simulink model "caishi1_3"  (R2022b)
settings: Solver=VariableStepAuto  StartTime=0.0  StopTime=100  RelTol=1e-3
values from neighbouring files (symbols this model uses):
  C = [1 0 0]    [caishi.m]
settings Model: Creator=HONOR  LastModifiedBy=acer
settings DebuggingCC: UnconnectedInputMsg=warning  UnconnectedOutputMsg=warning  UnconnectedLineMsg=warning
settings ModelReferenceCC: EnableRefExpFcnMdlSchedulingChecks=on
settings RTWCC: DLArmComputeVersion=19.05

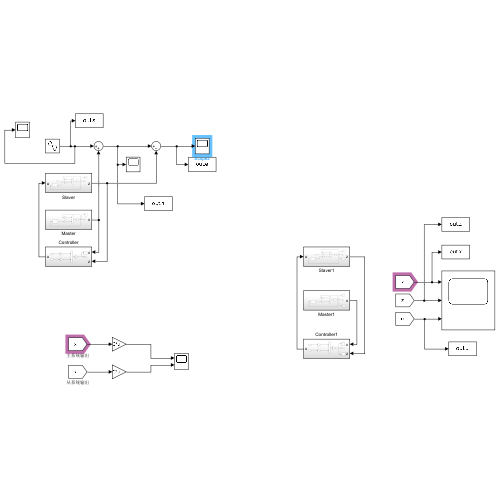
[thumbnail: Simulink's stored preview of the top-level diagram]
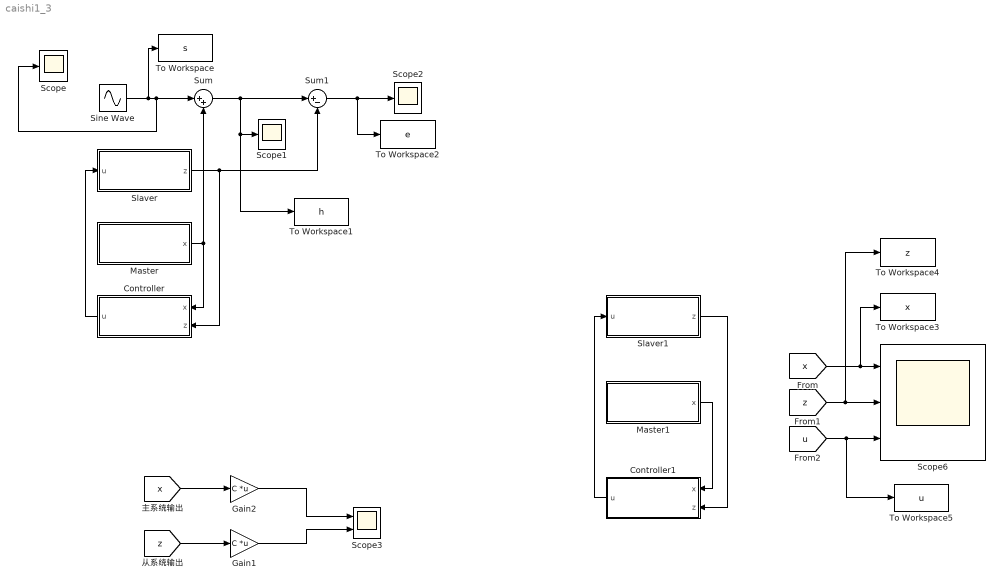
== system caishi1_3 ==
  Controller : Subsystem
  Controller1 : Subsystem
  Gain1 : Gain  Gain=C  Multiplication=Matrix(K*u)
  Gain2 : Gain  Gain=C  Multiplication=Matrix(K*u)
  Master : Subsystem
  Master1 : Subsystem
  Scope : Scope
  Scope1 : Scope
  Scope2 : Scope
  Scope3 : Scope  NumInputPorts=2
  Scope6 : Scope  NumInputPorts=3
  Sine Wave : Sin  SampleTime=0
  Slaver : Subsystem
  Slaver1 : Subsystem
  Sum : Sum  Inputs=|++
  Sum1 : Sum  Inputs=|+-
  To Workspace : ToWorkspace  VariableName=s  SaveFormat=Structure With Time  SampleTime=-1
  To Workspace1 : ToWorkspace  VariableName=h  SaveFormat=Structure With Time  SampleTime=-1
  To Workspace2 : ToWorkspace  VariableName=e  SaveFormat=Structure With Time  SampleTime=-1
  To Workspace3 : ToWorkspace  VariableName=x  SaveFormat=Structure With Time  SampleTime=-1
  To Workspace4 : ToWorkspace  VariableName=z  SaveFormat=Structure With Time  SampleTime=-1
  To Workspace5 : ToWorkspace  VariableName=u  SaveFormat=Structure With Time  SampleTime=-1
  wires:
  Controller/1(u) -> Slaver/1(u)
  Master/1(x) -> Controller/1(x), Sum/2
  Slaver/1(z) -> Sum1/2, Controller/2(z)
  Sine Wave/1 -> To Workspace/1, Scope/1, Sum/1
  Sum/1 -> Sum1/1, To Workspace1/1, Scope1/1
  Sum1/1 -> Scope2/1, To Workspace2/1
  Controller1/1(u) -> Slaver1/1(u)
  Master1/1(x) -> Controller1/1(x)
  Slaver1/1(z) -> Controller1/2(z)
  [z] -> To Workspace4/1, Scope6/2
  [u] -> To Workspace5/1, Scope6/3
  [x] -> To Workspace3/1, Scope6/1
  [x] -> Gain2/1
  [z] -> Gain1/1
  Gain2/1 -> Scope3/1
  Gain1/1 -> Scope3/2

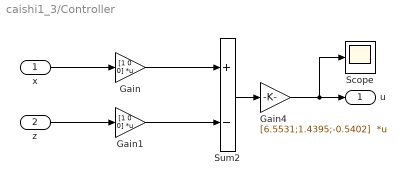
== system caishi1_3/Controller ==
  x : Inport
  z : Inport  Port=2
  Gain : Gain  Gain=[1 0 0]  Multiplication=Matrix(K*u)
  Gain1 : Gain  Gain=[1 0 0]  Multiplication=Matrix(K*u)
  Gain4 : Gain  Gain=[6.5531;1.4395;-0.5402]  Multiplication=Matrix(K*u)
  Scope : Scope
  Sum2 : Sum  Inputs=+-
  u : Outport
  wires:
  Gain1/1 -> Sum2/2
  Gain/1 -> Sum2/1
  Sum2/1 -> Gain4/1
  Gain4/1 -> Scope/1, u/1
  x/1 -> Gain/1
  z/1 -> Gain1/1

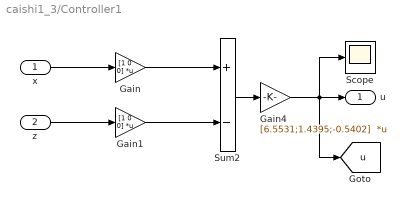
== system caishi1_3/Controller1 ==
  x : Inport
  z : Inport  Port=2
  Gain : Gain  Gain=[1 0 0]  Multiplication=Matrix(K*u)
  Gain1 : Gain  Gain=[1 0 0]  Multiplication=Matrix(K*u)
  Gain4 : Gain  Gain=[6.5531;1.4395;-0.5402]  Multiplication=Matrix(K*u)
  Scope : Scope
  Sum2 : Sum  Inputs=+-
  u : Outport
  tag scope: u=global
  wires:
  Gain1/1 -> Sum2/2
  Gain/1 -> Sum2/1
  Sum2/1 -> Gain4/1
  Gain4/1 -> [u], Scope/1, u/1
  x/1 -> Gain/1
  z/1 -> Gain1/1

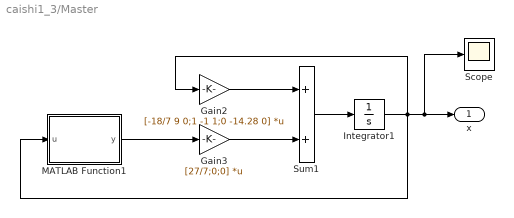
== system caishi1_3/Master ==
  Gain2 : Gain  Gain=[-18/7 9 0;1 -1 1;0 -14.28 0]  Multiplication=Matrix(K*u)
  Gain3 : Gain  Gain=[27/7;0;0]  Multiplication=Matrix(K*u)
  Integrator1 : Integrator  InitialCondition=[-0.1,0.1,0.2]
  MATLAB Function1 : MATLAB Function  TreatAsAtomicUnit=on
  Scope : Scope
  Sum1 : Sum
  x : Outport
  wires:
  Sum1/1 -> Integrator1/1
  Integrator1/1 -> Gain2/1, MATLAB Function1/1(u), Scope/1, x/1
  Gain2/1 -> Sum1/1
  Gain3/1 -> Sum1/2
  MATLAB Function1/1(y) -> Gain3/1

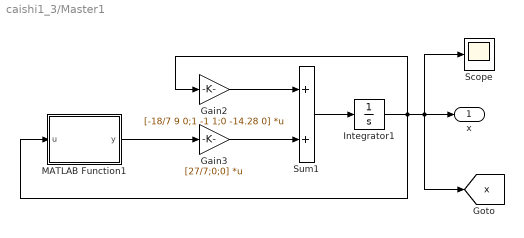
== system caishi1_3/Master1 ==
  Gain2 : Gain  Gain=[-18/7 9 0;1 -1 1;0 -14.28 0]  Multiplication=Matrix(K*u)
  Gain3 : Gain  Gain=[27/7;0;0]  Multiplication=Matrix(K*u)
  Integrator1 : Integrator  InitialCondition=[-0.1,0.1,0.2]
  MATLAB Function1 : MATLAB Function  TreatAsAtomicUnit=on
  Scope : Scope
  Sum1 : Sum
  x : Outport
  tag scope: x=global
  wires:
  Sum1/1 -> Integrator1/1
  Integrator1/1 -> Gain2/1, MATLAB Function1/1(u), [x], Scope/1, x/1
  Gain2/1 -> Sum1/1
  Gain3/1 -> Sum1/2
  MATLAB Function1/1(y) -> Gain3/1

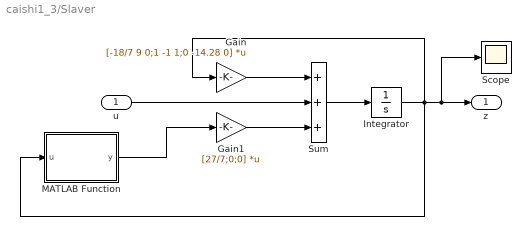
== system caishi1_3/Slaver ==
  u : Inport
  Gain : Gain  Gain=[-18/7 9 0;1 -1 1;0 -14.28 0]  Multiplication=Matrix(K*u)
  Gain1 : Gain  Gain=[27/7;0;0]  Multiplication=Matrix(K*u)
  Integrator : Integrator  InitialCondition=[1,2,3]
  MATLAB Function : MATLAB Function  TreatAsAtomicUnit=on
  Scope : Scope
  Sum : Sum  Inputs=+++
  z : Outport
  wires:
  Gain1/1 -> Sum/3
  Integrator/1 -> Gain/1, MATLAB Function/1(u), Scope/1, z/1
  Sum/1 -> Integrator/1
  Gain/1 -> Sum/1
  u/1 -> Sum/2
  MATLAB Function/1(y) -> Gain1/1

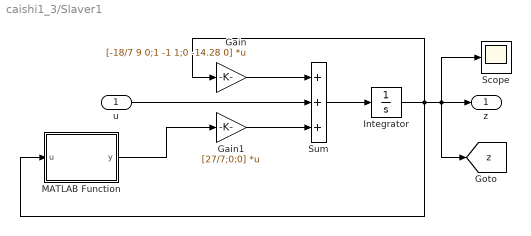
== system caishi1_3/Slaver1 ==
  u : Inport
  Gain : Gain  Gain=[-18/7 9 0;1 -1 1;0 -14.28 0]  Multiplication=Matrix(K*u)
  Gain1 : Gain  Gain=[27/7;0;0]  Multiplication=Matrix(K*u)
  Integrator : Integrator  InitialCondition=[1,2,3]
  MATLAB Function : MATLAB Function  TreatAsAtomicUnit=on
  Scope : Scope
  Sum : Sum  Inputs=+++
  z : Outport
  tag scope: z=global
  wires:
  Gain1/1 -> Sum/3
  Integrator/1 -> Gain/1, MATLAB Function/1(u), [z], Scope/1, z/1
  Sum/1 -> Integrator/1
  Gain/1 -> Sum/1
  u/1 -> Sum/2
  MATLAB Function/1(y) -> Gain1/1

== matlab function caishi1_3/Slaver/MATLAB Function ==
  data: u input; y output
function y = fcn(u)
y=(abs(u(1)+1)-abs(u(1)-1))/2;

== matlab function caishi1_3/Slaver1/MATLAB Function ==
  data: u input; y output
function y = fcn(u)
y=(abs(u(1)+1)-abs(u(1)-1))/2;

== matlab function caishi1_3/Master1/MATLAB Function1 ==
  data: u input; y output
function y = fcn(u)
y=(abs(u(1)+1)-abs(u(1)-1))/2;

== matlab function caishi1_3/Master/MATLAB Function1 ==
  data: u input; y output
function y = fcn(u)
y=(abs(u(1)+1)-abs(u(1)-1))/2;
